simulink model "secondorder"  (R2022b)
settings: Solver=VariableStepAuto  StartTime=0.0  StopTime=2  RelTol=1e-3
settings Model: Creator=Asus  LastModifiedBy=Asus

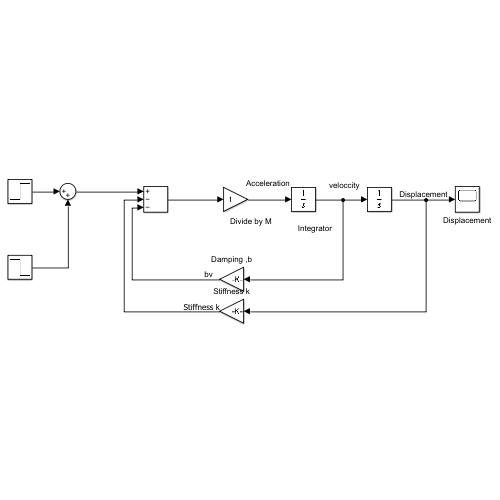
[thumbnail: Simulink's stored preview of the top-level diagram]
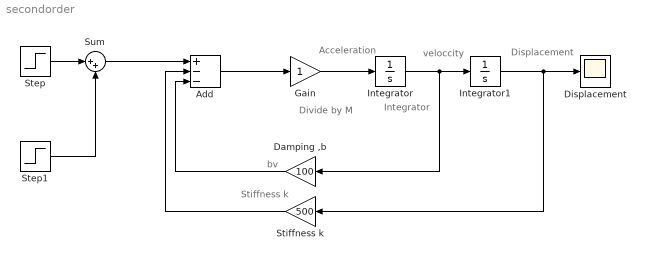
== system secondorder ==
  note: Stiffness k
  note: Displacement
  note: Integrator
  note: Divide by M
  note: veloccity
  note: bv
  note: Acceleration
  Add : Sum  Inputs=+--
  Damping ,b : Gain  Gain=100
  Displacement : Scope
  Gain : Gain
  Integrator : Integrator
  Integrator1 : Integrator
  Step : Step  Time=0  SampleTime=0
  Step1 : Step  After=-5  SampleTime=0
  Stiffness k : Gain  Gain=500
  Sum : Sum  Inputs=|++
  wires:
  Integrator/1 -> Integrator1/1, Damping ,b/1
  Gain/1 -> Integrator/1
  Integrator1/1 -> Stiffness k/1, Displacement/1
  Damping ,b/1 -> Add/3
  Stiffness k/1 -> Add/2
  Add/1 -> Gain/1
  Step/1 -> Sum/1
  Step1/1 -> Sum/2
  Sum/1 -> Add/1
